simulink model "modelo_ma"  (R2023a)
settings: Solver=VariableStepAuto  StartTime=0.0  StopTime=1000  RelTol=1e-3
libraries: cstblocks x1
settings Model: Creator=vitor  LastModifiedBy=vitor

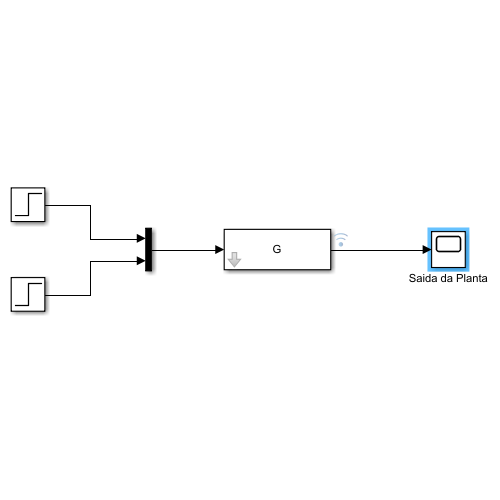
[thumbnail: Simulink's stored preview of the top-level diagram]
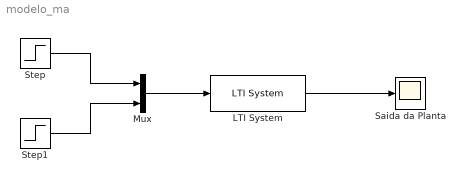
== system modelo_ma ==
  LTI System : cstblocks/LTI System  sys=G  IC=[]
  Mux : Mux  Inputs=2
  Saida da Planta : Scope
  Step : Step  SampleTime=0
  Step1 : Step  SampleTime=0
  wires:
  LTI System/1 -> Saida da Planta/1
  Mux/1 -> LTI System/1
  Step/1 -> Mux/1
  Step1/1 -> Mux/2
